simulink model "power_aircraft_distribution_mexido_2016_V4"  (R2016a)
settings: Solver=ode23t  StartTime=72.95  StopTime=73.6  MaxStep=0.01  RelTol=0.5e-4  AbsTol=0.5e-4
PreLoadFcn:
  | % -- Recommended Settings --
  | %
  | %  Simulink:
  | %      Solver: Ode23t
  | %      Relative tolerance = 1e-3
  | %       Max step size = 0.2
  | %
  | %  Powergui:
  |          Ts = 1e-07; % (discrete electrical model)
  | %
  | %  Control systems:
  |          Ts_control = 10*Ts; % (discrete control system)
  | %
  | % ----------------------------------
undefined symbols (not defined in the file or in its folder): C, D1, Delta, L, sigbuilder_block, tb1, tb2, tb3
libraries: powerlib x79, dsparch4 x12, simulink x6, sps_avr x1, powerlib_meascontrol x1
(part 1 of 2)
settings Model: Creator=Joao  LastModifiedBy=Joao
settings DataIOCC: InitialState=xFinal  LimitDataPoints=on  SaveCompleteFinalSimState=on
settings DebuggingCC: AllowSymbolicDim=off
settings ConfigComp: CovModelRefEnable=Off  CovSFcnEnable=off

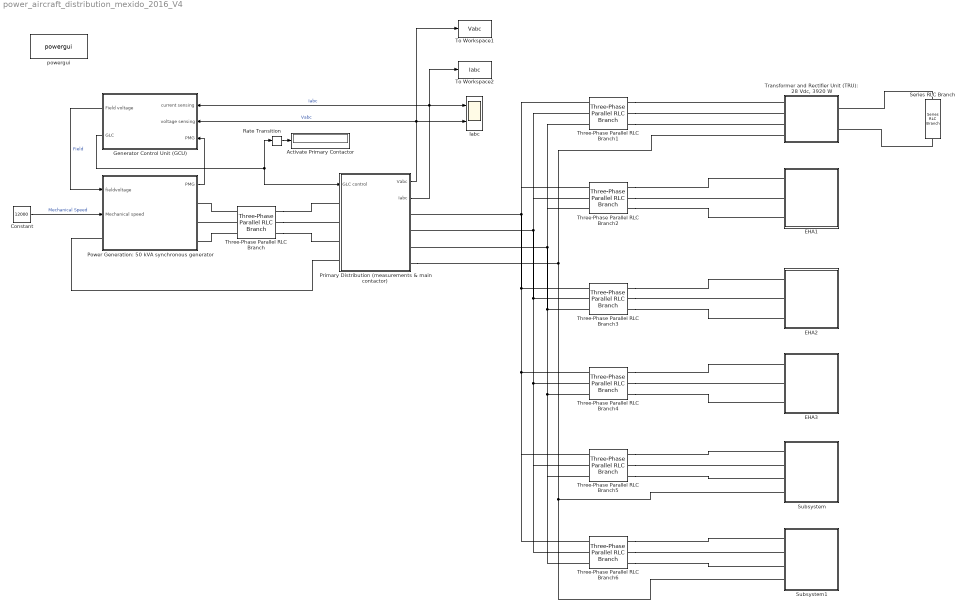
== system power_aircraft_distribution_mexido_2016_V4 ==
  Activate Primary Contactor : Display
      settings: SampleTime=1e-2
  Constant : Constant  Value=12000
  EHA1 : Subsystem
  EHA2 : Subsystem
  EHA3 : Subsystem
  Generator Control Unit (GCU) : Subsystem
      mask Display: image(imread('power_aircraft_distribution_GCU.jpg','jpg'))
  Iabc : Scope  NumInputPorts=2
  Power Generation: 50 kVA synchronous generator : Subsystem
      mask Display: image(imread('power_aircraft_distribution_APU_Generator.jpg','jpg'))
  Primary Distribution (measurements & main contactor) : Subsystem
  Rate Transition : RateTransition  OutPortSampleTimeOpt=Inherit  OutPortSampleTime=Ts
  Series RLC Branch : powerlib/Elements/Series RLC Branch  LConnTagsString=__new0  RConnTagsString=__new0  BranchType=R  Resistance=0.2  Inductance=1e-3  SetiL0=off  InitialCurrent=0  Capacitance=1e-6  Setx0=off  InitialVoltage=0  Measurements=None
  Subsystem : Subsystem
  Subsystem1 : Subsystem
  Three-Phase Parallel RLC Branch : powerlib/Elements/Three-Phase Parallel RLC Branch  LConnTagsString=A|B|C  RConnTagsString=A|B|C  BranchType=RL  Resistance=0.00047*10  Inductance=5e-6  Capacitance=0  Measurements=None
  Three-Phase Parallel RLC Branch1 : powerlib/Elements/Three-Phase Parallel RLC Branch  LConnTagsString=A|B|C  RConnTagsString=A|B|C  BranchType=RL  Resistance=0.00228*3  Inductance=5e-7  Capacitance=0  Measurements=None
  Three-Phase Parallel RLC Branch2 : powerlib/Elements/Three-Phase Parallel RLC Branch  LConnTagsString=A|B|C  RConnTagsString=A|B|C  BranchType=RL  Resistance=0.00227*15  Inductance=3e-6  Capacitance=0  Measurements=None
  Three-Phase Parallel RLC Branch3 : powerlib/Elements/Three-Phase Parallel RLC Branch  LConnTagsString=A|B|C  RConnTagsString=A|B|C  BranchType=RL  Resistance=0.00227*17.5  Inductance=3e-6  Capacitance=0  Measurements=None
  Three-Phase Parallel RLC Branch4 : powerlib/Elements/Three-Phase Parallel RLC Branch  LConnTagsString=A|B|C  RConnTagsString=A|B|C  BranchType=RL  Resistance=0.00227*20  Inductance=3e-6  Capacitance=0  Measurements=None
  Three-Phase Parallel RLC Branch5 : powerlib/Elements/Three-Phase Parallel RLC Branch  LConnTagsString=A|B|C  RConnTagsString=A|B|C  BranchType=RL  Resistance=0.00228*20  Inductance=10e-6  Capacitance=0  Measurements=None
  Three-Phase Parallel RLC Branch6 : powerlib/Elements/Three-Phase Parallel RLC Branch  LConnTagsString=A|B|C  RConnTagsString=A|B|C  BranchType=RL  Resistance=0.00228*8  Inductance=5e-6  Capacitance=0  Measurements=None
  To Workspace1 : ToWorkspace  VariableName=Vabc  SaveFormat=Structure With Time  SampleTime=-1
  To Workspace2 : ToWorkspace  VariableName=Iabc  SaveFormat=Structure With Time  SampleTime=-1
  "Transformer and Rectifier Unit (TRU): 28 Vdc, 3920 W" : Subsystem
      mask Display: image(imread('power_aircraft_distribution_TRU.jpg','jpg'))
  powergui : powerlib/powergui  Priority=1  SimulationMode=Discrete  SolverType=Tustin/Backward Euler (TBE)  SampleTime=Ts  frequency=60  SPID=off  DisableSnubberDevices=off  DisableRonSwitches=off  DisableVfSwitches=off  SwTol=0  DisplayEquations=off  Interpol=off  ExternalGateDelay=off  methode=off  Ts=100  FunctionMessages=on  echomessages=off  HookPort=off  EnableUseOfTLC=off  x0status=blocks  frequencyindice=0  Pbase=100e6  ErrMax=1e-4  Iterations=50  UnitsV=kV  UnitsW=MW  buscounter=0  RestoreLinks=warning  ResistiveCurrentMeasurement=off  Frange=[0:2:500]  Ylog=off  Xlog=on  ShowGrid=off  save=off  variable=ZData  structure=0  ZoomFFT=off  StartTime=0.0  cycles=1  DisplayStyle=1  fundamental=60  FreqAxis=off  MaxFrequency=1000  frequencyindicesteady=1  RmsSteady=1  display=off
  wires:
  Power Generation: 50 kVA synchronous generator/1(PMG) -> Generator Control Unit (GCU)/3(PMG)
  Generator Control Unit (GCU)/1(Field voltage) -> Power Generation: 50 kVA synchronous generator/1(fieldvoltage)  "Field"
  Primary Distribution (measurements & main contactor)/1(Vabc) -> Generator Control Unit (GCU)/2(voltage sensing), To Workspace1/1, Iabc/2  "Vabc"
  Primary Distribution (measurements & main contactor)/2(Iabc) -> To Workspace2/1, Generator Control Unit (GCU)/1(current sensing), Iabc/1  "Iabc"
  Generator Control Unit (GCU)/2(GLC) -> Primary Distribution (measurements & main contactor)/1(GLC control), Rate Transition/1
  Constant/1 -> Power Generation: 50 kVA synchronous generator/2(Mechanical speed)  "Mechanical Speed"
  Rate Transition/1 -> Activate Primary Contactor/1
  connections:
  Three-Phase Parallel RLC Branch6/LConn1 -- Three-Phase Parallel RLC Branch5/LConn1 -- Three-Phase Parallel RLC Branch4/LConn1 -- Three-Phase Parallel RLC Branch3/LConn1 -- Primary Distribution (measurements & main contactor)/RConn1 -- Three-Phase Parallel RLC Branch2/LConn1 -- Three-Phase Parallel RLC Branch1/LConn1
  Primary Distribution (measurements & main contactor)/RConn4 -- "Transformer and Rectifier Unit (TRU): 28 Vdc, 3920 W"/LConn4 -- Subsystem1/LConn4 -- Subsystem/LConn4
  Three-Phase Parallel RLC Branch6/LConn3 -- Three-Phase Parallel RLC Branch5/LConn3 -- Three-Phase Parallel RLC Branch4/LConn3 -- Three-Phase Parallel RLC Branch3/LConn3 -- Primary Distribution (measurements & main contactor)/RConn3 -- Three-Phase Parallel RLC Branch2/LConn3 -- Three-Phase Parallel RLC Branch1/LConn3
  Three-Phase Parallel RLC Branch6/LConn2 -- Three-Phase Parallel RLC Branch5/LConn2 -- Three-Phase Parallel RLC Branch4/LConn2 -- Three-Phase Parallel RLC Branch3/LConn2 -- Primary Distribution (measurements & main contactor)/RConn2 -- Three-Phase Parallel RLC Branch2/LConn2 -- Three-Phase Parallel RLC Branch1/LConn2
  Three-Phase Parallel RLC Branch/RConn2 -- Primary Distribution (measurements & main contactor)/LConn2
  Three-Phase Parallel RLC Branch/LConn2 -- Power Generation: 50 kVA synchronous generator/RConn2
  Three-Phase Parallel RLC Branch/LConn1 -- Power Generation: 50 kVA synchronous generator/RConn1
  Three-Phase Parallel RLC Branch/LConn3 -- Power Generation: 50 kVA synchronous generator/RConn3
  Three-Phase Parallel RLC Branch/RConn1 -- Primary Distribution (measurements & main contactor)/LConn1
  Three-Phase Parallel RLC Branch/RConn3 -- Primary Distribution (measurements & main contactor)/LConn3
  Power Generation: 50 kVA synchronous generator/LConn1 -- Primary Distribution (measurements & main contactor)/LConn4
  Series RLC Branch/RConn1 -- "Transformer and Rectifier Unit (TRU): 28 Vdc, 3920 W"/RConn2
  Series RLC Branch/LConn1 -- "Transformer and Rectifier Unit (TRU): 28 Vdc, 3920 W"/RConn1
  Three-Phase Parallel RLC Branch1/RConn1 -- "Transformer and Rectifier Unit (TRU): 28 Vdc, 3920 W"/LConn1
  Three-Phase Parallel RLC Branch1/RConn2 -- "Transformer and Rectifier Unit (TRU): 28 Vdc, 3920 W"/LConn2
  Three-Phase Parallel RLC Branch1/RConn3 -- "Transformer and Rectifier Unit (TRU): 28 Vdc, 3920 W"/LConn3
  Three-Phase Parallel RLC Branch5/RConn1 -- Subsystem/LConn1
  Three-Phase Parallel RLC Branch5/RConn2 -- Subsystem/LConn2
  Three-Phase Parallel RLC Branch5/RConn3 -- Subsystem/LConn3
  Three-Phase Parallel RLC Branch6/RConn1 -- Subsystem1/LConn1
  Three-Phase Parallel RLC Branch6/RConn2 -- Subsystem1/LConn2
  Three-Phase Parallel RLC Branch6/RConn3 -- Subsystem1/LConn3
  Three-Phase Parallel RLC Branch2/RConn1 -- EHA1/LConn1
  Three-Phase Parallel RLC Branch2/RConn2 -- EHA1/LConn2
  Three-Phase Parallel RLC Branch2/RConn3 -- EHA1/LConn3
  Three-Phase Parallel RLC Branch3/RConn1 -- EHA2/LConn1
  Three-Phase Parallel RLC Branch3/RConn2 -- EHA2/LConn2
  Three-Phase Parallel RLC Branch3/RConn3 -- EHA2/LConn3
  Three-Phase Parallel RLC Branch4/RConn1 -- EHA3/LConn1
  Three-Phase Parallel RLC Branch4/RConn2 -- EHA3/LConn2
  Three-Phase Parallel RLC Branch4/RConn3 -- EHA3/LConn3

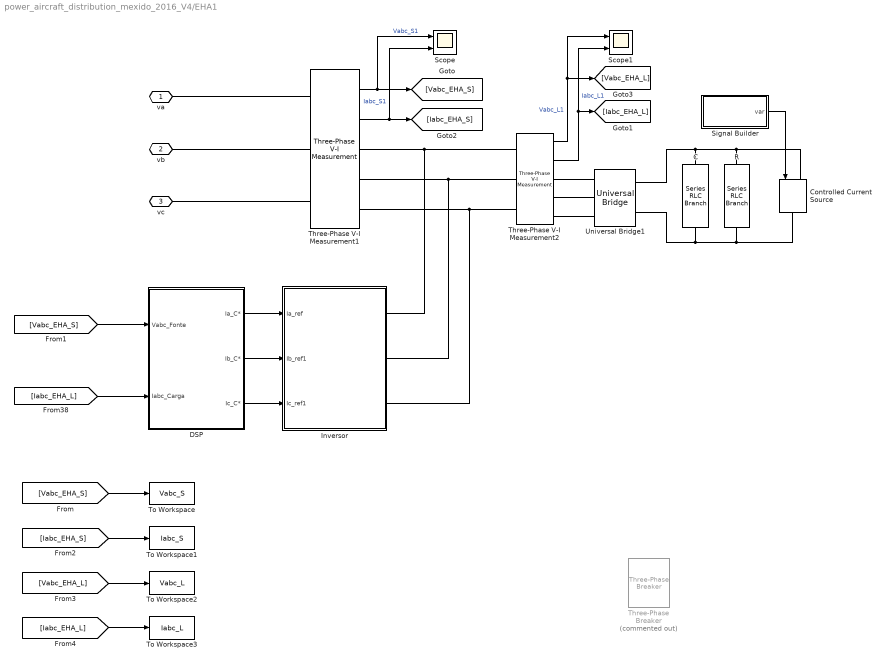
== system power_aircraft_distribution_mexido_2016_V4/EHA1 ==
  C : powerlib/Elements/Series RLC Branch  LConnTagsString=__new0  RConnTagsString=__new0  BranchType=C  Resistance=1  Inductance=1e-3  SetiL0=off  InitialCurrent=0  Capacitance=1e-7  Setx0=off  InitialVoltage=0  Measurements=None
  Controlled Current Source : powerlib/Electrical Sources/Controlled Current Source  Initialize=on  Source_Type=AC  Amplitude=0  Phase=0  Frequency=0  Measurements=None
  DSP : Subsystem
  Inversor : Subsystem
  R : powerlib/Elements/Series RLC Branch  LConnTagsString=__new0  RConnTagsString=__new0  BranchType=R  Resistance=400  Inductance=1e-3  SetiL0=off  InitialCurrent=0  Capacitance=1e-10  Setx0=off  InitialVoltage=0  Measurements=None
  Scope : Scope  NumInputPorts=2
  Scope1 : Scope  NumInputPorts=2
  Signal Builder : Subsystem  Tag=STV Subsys  LoadFcn=sigbuilder_block('load',[437.6 199.2 550.4 400 ]);  StartFcn=sigbuilder_block('start');  StopFcn=sigbuilder_block('stop');  ClipboardFcn=sigbuilder_block('clipboard');  mask(Sigbuilder block){}
      mask help: Simulink:masks:SigbuilderBlock_MD
      mask init:
      | if ~strcmp(get_param(bdroot(gcbh),'SimulationStatus'),'stopped') tuvar = sigbuilder_block('maskInit'); end
      settings: CopyFcn=sigbuilder_block('copy');  DeleteFcn=sigbuilder_block('delete');  ModelCloseFcn=sigbuilder_block('modelClose');  PreSaveFcn=sigbuilder_block('preSave');  PauseFcn=sigbuilder_block('pause');  ContinueFcn=sigbuilder_block('continue');  NameChangeFcn=sigbuilder_block('namechange');  OpenFcn=sigbuilder_block('open',[437.6 199.2 550.4 400 ]);  CloseFcn=sigbuilder_block('close');
      mask Display: plot(0, 0, 100, 100,[2, 2, 32, 32, 2], [68, 8, 8, 68, 68],[32, 2], [38, 38], [32, 19, 2],[53, 60, 44], [32, 17, 17, 2],[16, 16, 31, 31]);txt = getActiveGroup(gcbh);text(2, 100, txt,'verticalAlignment', 'top');
  Three-Phase V-I Measurement1 : powerlib/Measurements/Three-Phase V-I Measurement  VoltageMeasurement=phase-to-ground  SetLabelV=off  LabelV=Vabc_EHA1_S  Vpu=off  VpuLL=off  CurrentMeasurement=yes  SetLabelI=off  LabelI=Iabc_EHA1_S  Ipu=off  Pbase=100e6  Vbase=500e3  OutputType=Complex  PhasorSimulation=off  PSBequivalent=0
  Three-Phase V-I Measurement2 : powerlib/Measurements/Three-Phase V-I Measurement  VoltageMeasurement=phase-to-ground  SetLabelV=off  LabelV=Vabc_EHA1_S  Vpu=off  VpuLL=off  CurrentMeasurement=yes  SetLabelI=off  LabelI=Iabc_EHA1_S  Ipu=off  Pbase=100e6  Vbase=500e3  OutputType=Complex  PhasorSimulation=off  PSBequivalent=0
  Three-Phase Breaker : powerlib/Elements/Three-Phase Breaker  Commented=on  InitialState=open  SwitchA=on  SwitchB=on  SwitchC=on  SwitchTimes=tb1  External=off  BreakerResistance=1e-3  SnubberResistance=1e6  SnubberCapacitance=inf  Measurements=None
  To Workspace : ToWorkspace  VariableName=Vabc_S  SaveFormat=Structure With Time  SampleTime=-1
  To Workspace1 : ToWorkspace  VariableName=Iabc_S  SaveFormat=Structure With Time  SampleTime=-1
  To Workspace2 : ToWorkspace  VariableName=Vabc_L  SaveFormat=Structure With Time  SampleTime=-1
  To Workspace3 : ToWorkspace  VariableName=Iabc_L  SaveFormat=Structure With Time  SampleTime=-1
  Universal Bridge1 : powerlib/Power Electronics/Universal Bridge  Arms=3  SnubberResistance=1e5  SnubberCapacitance=inf  Device=Diodes  Ron=1e-9  Lon=0  ForwardVoltages="[  0  0  ]"  ForwardVoltage=0  GTOparameters=[ 10e-6 , 20e-6 ]  IGBTparameters=[ 1e-6 , 2e-6 ]  Measurements=None  Measurements_2=None  converterType=Rectifier
  va : PMIOPort  Port=1  Side=Left
  vb : PMIOPort  Port=2  Side=Left
  vc : PMIOPort  Port=3  Side=Left
  wires:
  Signal Builder/1(var) -> Controlled Current Source/1
  Three-Phase V-I Measurement1/1 -> [Vabc_EHA_S], Scope/1  "Vabc_S1"
  Three-Phase V-I Measurement1/2 -> [Iabc_EHA_S], Scope/2  "Iabc_S1"
  Three-Phase V-I Measurement2/1 -> [Vabc_EHA_L], Scope1/1  "Vabc_L1"
  Three-Phase V-I Measurement2/2 -> [Iabc_EHA_L], Scope1/2  "Iabc_L1"
  [Vabc_EHA_S] -> DSP/1(Vabc_Fonte)
  [Iabc_EHA_L] -> DSP/2(Iabc_Carga)
  DSP/1(Ia_C*) -> Inversor/1(Ia_ref)
  DSP/2(Ib_C*) -> Inversor/2(Ib_ref1)
  DSP/3(Ic_C*) -> Inversor/3(Ic_ref1)
  [Vabc_EHA_S] -> To Workspace/1
  [Iabc_EHA_S] -> To Workspace1/1
  [Vabc_EHA_L] -> To Workspace2/1
  [Iabc_EHA_L] -> To Workspace3/1
  connections:
  R/LConn1 -- Controlled Current Source/LConn1 -- Universal Bridge1/RConn1 -- C/LConn1
  Controlled Current Source/RConn1 -- R/RConn1 -- Universal Bridge1/RConn2 -- C/RConn1
  Three-Phase V-I Measurement2/RConn2 -- Universal Bridge1/LConn2
  Three-Phase V-I Measurement2/RConn1 -- Universal Bridge1/LConn1
  Three-Phase V-I Measurement2/RConn3 -- Universal Bridge1/LConn3
  Three-Phase V-I Measurement1/RConn3 -- Three-Phase V-I Measurement2/LConn3 -- Inversor/RConn3
  Three-Phase V-I Measurement2/LConn1 -- Three-Phase V-I Measurement1/RConn1 -- Inversor/RConn1
  Three-Phase V-I Measurement2/LConn2 -- Three-Phase V-I Measurement1/RConn2 -- Inversor/RConn2
  vb/RConn1 -- Three-Phase V-I Measurement1/LConn2
  vc/RConn1 -- Three-Phase V-I Measurement1/LConn3
  va/RConn1 -- Three-Phase V-I Measurement1/LConn1

== system power_aircraft_distribution_mexido_2016_V4/EHA2 ==
  C : powerlib/Elements/Series RLC Branch  LConnTagsString=__new0  RConnTagsString=__new0  BranchType=C  Resistance=1  Inductance=1e-3  SetiL0=off  InitialCurrent=0  Capacitance=1e-7  Setx0=off  InitialVoltage=0  Measurements=None
  Controlled Current Source : powerlib/Electrical Sources/Controlled Current Source  Initialize=on  Source_Type=AC  Amplitude=0  Phase=0  Frequency=0  Measurements=None
  DSP : Subsystem
  Inversor : Subsystem
  R : powerlib/Elements/Series RLC Branch  LConnTagsString=__new0  RConnTagsString=__new0  BranchType=R  Resistance=400  Inductance=1e-3  SetiL0=off  InitialCurrent=0  Capacitance=1e-10  Setx0=off  InitialVoltage=0  Measurements=None
  Scope : Scope  NumInputPorts=2
  Scope1 : Scope  NumInputPorts=2
  Signal Builder : Subsystem  Tag=STV Subsys  LoadFcn=sigbuilder_block('load');  StartFcn=sigbuilder_block('start');  StopFcn=sigbuilder_block('stop');  ClipboardFcn=sigbuilder_block('clipboard');  mask(Sigbuilder block){}
      mask help: Simulink:masks:SigbuilderBlock_MD
      mask init:
      | if ~strcmp(get_param(bdroot(gcbh),'SimulationStatus'),'stopped') tuvar = sigbuilder_block('maskInit'); end
      settings: CopyFcn=sigbuilder_block('copy');  DeleteFcn=sigbuilder_block('delete');  ModelCloseFcn=sigbuilder_block('modelClose');  PreSaveFcn=sigbuilder_block('preSave');  PauseFcn=sigbuilder_block('pause');  ContinueFcn=sigbuilder_block('continue');  NameChangeFcn=sigbuilder_block('namechange');  OpenFcn=sigbuilder_block('open',[437.6 199.2 550.4 400 ]);  CloseFcn=sigbuilder_block('close');
      mask Display: plot(0, 0, 100, 100,[2, 2, 32, 32, 2], [68, 8, 8, 68, 68],[32, 2], [38, 38], [32, 19, 2],[53, 60, 44], [32, 17, 17, 2],[16, 16, 31, 31]);txt = getActiveGroup(gcbh);text(2, 100, txt,'verticalAlignment', 'top');
  Three-Phase V-I Measurement1 : powerlib/Measurements/Three-Phase V-I Measurement  VoltageMeasurement=phase-to-ground  SetLabelV=off  LabelV=Vabc_EHA1_S  Vpu=off  VpuLL=off  CurrentMeasurement=yes  SetLabelI=off  LabelI=Iabc_EHA1_S  Ipu=off  Pbase=100e6  Vbase=500e3  OutputType=Complex  PhasorSimulation=off  PSBequivalent=0
  Three-Phase V-I Measurement2 : powerlib/Measurements/Three-Phase V-I Measurement  VoltageMeasurement=phase-to-ground  SetLabelV=off  LabelV=Vabc_EHA1_S  Vpu=off  VpuLL=off  CurrentMeasurement=yes  SetLabelI=off  LabelI=Iabc_EHA1_S  Ipu=off  Pbase=100e6  Vbase=500e3  OutputType=Complex  PhasorSimulation=off  PSBequivalent=0
  Three-Phase Breaker : powerlib/Elements/Three-Phase Breaker  Commented=on  InitialState=open  SwitchA=on  SwitchB=on  SwitchC=on  SwitchTimes=tb2  External=off  BreakerResistance=1e-3  SnubberResistance=1e6  SnubberCapacitance=inf  Measurements=None
  Universal Bridge1 : powerlib/Power Electronics/Universal Bridge  Arms=3  SnubberResistance=1e5  SnubberCapacitance=inf  Device=Diodes  Ron=1e-9  Lon=0  ForwardVoltages="[  0  0  ]"  ForwardVoltage=0  GTOparameters=[ 10e-6 , 20e-6 ]  IGBTparameters=[ 1e-6 , 2e-6 ]  Measurements=None  Measurements_2=None  converterType=Rectifier
  va : PMIOPort  Port=1  Side=Left
  vb : PMIOPort  Port=2  Side=Left
  vc : PMIOPort  Port=3  Side=Left
  wires:
  Signal Builder/1(var) -> Controlled Current Source/1
  Three-Phase V-I Measurement1/1 -> [Vabc_EHA_S], Scope/1  "Vabc_S2"
  Three-Phase V-I Measurement1/2 -> Scope/2  "Iabc_S2"
  Three-Phase V-I Measurement2/1 -> Scope1/1  "Vabc_L2"
  Three-Phase V-I Measurement2/2 -> [Iabc_EHA_L], Scope1/2  "Iabc_L2"
  [Vabc_EHA_S] -> DSP/1(Vabc_Fonte)
  [Iabc_EHA_L] -> DSP/2(Iabc_Carga)
  DSP/1(Ia_C*) -> Inversor/1(Ia_ref)
  DSP/2(Ib_C*) -> Inversor/2(Ib_ref1)
  DSP/3(Ic_C*) -> Inversor/3(Ic_ref1)
  connections:
  R/LConn1 -- Controlled Current Source/LConn1 -- Universal Bridge1/RConn1 -- C/LConn1
  Controlled Current Source/RConn1 -- R/RConn1 -- Universal Bridge1/RConn2 -- C/RConn1
  Three-Phase V-I Measurement2/RConn2 -- Universal Bridge1/LConn2
  Three-Phase V-I Measurement2/RConn1 -- Universal Bridge1/LConn1
  Three-Phase V-I Measurement2/RConn3 -- Universal Bridge1/LConn3
  Three-Phase V-I Measurement1/RConn3 -- Three-Phase V-I Measurement2/LConn3 -- Inversor/RConn3
  Three-Phase V-I Measurement2/LConn1 -- Three-Phase V-I Measurement1/RConn1 -- Inversor/RConn1
  Three-Phase V-I Measurement2/LConn2 -- Three-Phase V-I Measurement1/RConn2 -- Inversor/RConn2
  Three-Phase V-I Measurement1/LConn2 -- vb/RConn1
  vc/RConn1 -- Three-Phase V-I Measurement1/LConn3
  va/RConn1 -- Three-Phase V-I Measurement1/LConn1

== system power_aircraft_distribution_mexido_2016_V4/EHA3 ==
  C : powerlib/Elements/Series RLC Branch  LConnTagsString=__new0  RConnTagsString=__new0  BranchType=C  Resistance=1  Inductance=1e-3  SetiL0=off  InitialCurrent=0  Capacitance=1e-7  Setx0=off  InitialVoltage=0  Measurements=None
  Controlled Current Source : powerlib/Electrical Sources/Controlled Current Source  Initialize=on  Source_Type=AC  Amplitude=0  Phase=0  Frequency=0  Measurements=None
  DSP : Subsystem
  Inversor : Subsystem
  R : powerlib/Elements/Series RLC Branch  LConnTagsString=__new0  RConnTagsString=__new0  BranchType=R  Resistance=400  Inductance=1e-3  SetiL0=off  InitialCurrent=0  Capacitance=1e-10  Setx0=off  InitialVoltage=0  Measurements=None
  Scope : Scope  NumInputPorts=2
  Scope1 : Scope  NumInputPorts=2
  Signal Builder : Subsystem  Tag=STV Subsys  LoadFcn=sigbuilder_block('load');  StartFcn=sigbuilder_block('start');  StopFcn=sigbuilder_block('stop');  ClipboardFcn=sigbuilder_block('clipboard');  mask(Sigbuilder block){}
      mask help: Simulink:masks:SigbuilderBlock_MD
      mask init:
      | if ~strcmp(get_param(bdroot(gcbh),'SimulationStatus'),'stopped') tuvar = sigbuilder_block('maskInit'); end
      settings: CopyFcn=sigbuilder_block('copy');  DeleteFcn=sigbuilder_block('delete');  ModelCloseFcn=sigbuilder_block('modelClose');  PreSaveFcn=sigbuilder_block('preSave');  PauseFcn=sigbuilder_block('pause');  ContinueFcn=sigbuilder_block('continue');  NameChangeFcn=sigbuilder_block('namechange');  OpenFcn=sigbuilder_block('open',[437.6 199.2 550.4 400 ]);  CloseFcn=sigbuilder_block('close');
      mask Display: plot(0, 0, 100, 100,[2, 2, 32, 32, 2], [68, 8, 8, 68, 68],[32, 2], [38, 38], [32, 19, 2],[53, 60, 44], [32, 17, 17, 2],[16, 16, 31, 31]);txt = getActiveGroup(gcbh);text(2, 100, txt,'verticalAlignment', 'top');
  Three-Phase V-I Measurement1 : powerlib/Measurements/Three-Phase V-I Measurement  VoltageMeasurement=phase-to-ground  SetLabelV=off  LabelV=Vabc_EHA1_S  Vpu=off  VpuLL=off  CurrentMeasurement=yes  SetLabelI=off  LabelI=Iabc_EHA1_S  Ipu=off  Pbase=100e6  Vbase=500e3  OutputType=Complex  PhasorSimulation=off  PSBequivalent=0
  Three-Phase V-I Measurement2 : powerlib/Measurements/Three-Phase V-I Measurement  VoltageMeasurement=phase-to-ground  SetLabelV=off  LabelV=Vabc_EHA1_S  Vpu=off  VpuLL=off  CurrentMeasurement=yes  SetLabelI=off  LabelI=Iabc_EHA1_S  Ipu=off  Pbase=100e6  Vbase=500e3  OutputType=Complex  PhasorSimulation=off  PSBequivalent=0
  Three-Phase Breaker : powerlib/Elements/Three-Phase Breaker  Commented=on  InitialState=open  SwitchA=on  SwitchB=on  SwitchC=on  SwitchTimes=tb3  External=off  BreakerResistance=1e-3  SnubberResistance=1e6  SnubberCapacitance=inf  Measurements=None
  Universal Bridge1 : powerlib/Power Electronics/Universal Bridge  Arms=3  SnubberResistance=1e5  SnubberCapacitance=inf  Device=Diodes  Ron=1e-9  Lon=0  ForwardVoltages="[  0  0  ]"  ForwardVoltage=0  GTOparameters=[ 10e-6 , 20e-6 ]  IGBTparameters=[ 1e-6 , 2e-6 ]  Measurements=None  Measurements_2=None  converterType=Rectifier
  va : PMIOPort  Port=1  Side=Left
  vb : PMIOPort  Port=2  Side=Left
  vc : PMIOPort  Port=3  Side=Left
  wires:
  Signal Builder/1(var) -> Controlled Current Source/1
  Three-Phase V-I Measurement1/1 -> [Vabc_EHA_S], Scope/1  "Vabc_S3"
  Three-Phase V-I Measurement1/2 -> Scope/2  "Iabc_S3"
  Three-Phase V-I Measurement2/1 -> Scope1/1  "Vabc_L3"
  Three-Phase V-I Measurement2/2 -> [Iabc_EHA_L], Scope1/2  "Iabc_L3"
  [Vabc_EHA_S] -> DSP/1(Vabc_Fonte)
  [Iabc_EHA_L] -> DSP/2(Iabc_Carga)
  DSP/1(Ia_C*) -> Inversor/1(Ia_ref)
  DSP/2(Ib_C*) -> Inversor/2(Ib_ref1)
  DSP/3(Ic_C*) -> Inversor/3(Ic_ref1)
  connections:
  R/LConn1 -- Controlled Current Source/LConn1 -- Universal Bridge1/RConn1 -- C/LConn1
  Controlled Current Source/RConn1 -- R/RConn1 -- Universal Bridge1/RConn2 -- C/RConn1
  Three-Phase V-I Measurement2/RConn2 -- Universal Bridge1/LConn2
  Three-Phase V-I Measurement2/RConn1 -- Universal Bridge1/LConn1
  Three-Phase V-I Measurement2/RConn3 -- Universal Bridge1/LConn3
  Three-Phase V-I Measurement1/RConn3 -- Three-Phase V-I Measurement2/LConn3 -- Inversor/RConn3
  Three-Phase V-I Measurement2/LConn1 -- Three-Phase V-I Measurement1/RConn1 -- Inversor/RConn1
  Three-Phase V-I Measurement2/LConn2 -- Three-Phase V-I Measurement1/RConn2 -- Inversor/RConn2
  vc/RConn1 -- Three-Phase V-I Measurement1/LConn3
  va/RConn1 -- Three-Phase V-I Measurement1/LConn1
  vb/RConn1 -- Three-Phase V-I Measurement1/LConn2

== system power_aircraft_distribution_mexido_2016_V4/Generator Control Unit (GCU) ==
  current sensing : Inport
  voltage sensing : Inport  Port=2
  PMG : Inport  Port=3
  Demux : Demux  Outputs=3
  Excitation System : sps_avr/Excitation System  tr=20e-3  reg=[ 300, 0.001 ]  exc=[ 1, 0 ]  tgr=[ 0, 0 ]  damp=[ 0.001, 0.1 ]  sat=[ 0, 0 ]  lim=[ -2, 2, 0 ]  v0=[1 0]
  Gain : Gain  Gain=2
  Integrator : Integrator
  PU_SI : Gain  Gain=200
  Rad_Rpm : Gain  Gain=30/pi
  Relay : Relay  OnSwitchValue=9000  OffSwitchValue=8900
  SI_PU : Gain  Gain=1/(115*sqrt(2))
  Terminator1 : Terminator
  Terminator2 : Terminator
  Vref : Constant
  abc to dq0 : powerlib_meascontrol/Transformations/abc to dq0  Alignment=90 degrees behind phase A axis
  threshold3 : Constant  Value=0
  Field voltage : Outport
  GLC : Outport  Port=2
  wires:
  Relay/1 -> GLC/1
  Demux/3 -> Terminator2/1
  current sensing/1 -> Terminator1/1
  threshold3/1 -> Excitation System/4
  Vref/1 -> Excitation System/1
  Rad_Rpm/1 -> Relay/1
  PU_SI/1 -> Field voltage/1
  Excitation System/1 -> PU_SI/1
  SI_PU/1 -> abc to dq0/1
  Demux/2 -> Excitation System/3
  Demux/1 -> Excitation System/2
  abc to dq0/1 -> Demux/1
  Integrator/1 -> Gain/1
  voltage sensing/1 -> SI_PU/1
  PMG/1 -> Rad_Rpm/1, Integrator/1
  Gain/1 -> abc to dq0/2

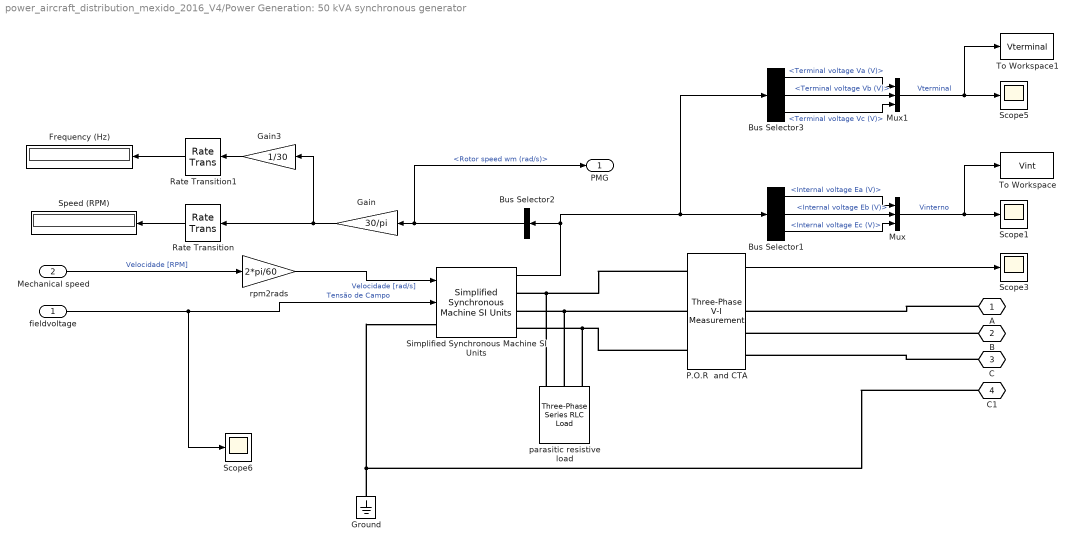
== system power_aircraft_distribution_mexido_2016_V4/Power Generation: 50 kVA synchronous generator ==
  fieldvoltage : Inport
  Mechanical speed : Inport  Port=2
  Bus Selector1 : BusSelector  OutputSignals=Internal voltage Ea (V),Internal voltage Eb (V),Internal voltage Ec (V)
  Bus Selector2 : BusSelector  OutputSignals=Rotor speed wm (rad/s)
  Bus Selector3 : BusSelector  OutputSignals=Terminal voltage Va (V),Terminal voltage Vb (V),Terminal voltage Vc (V)
  Frequency (Hz) : Display
      settings: SampleTime=1e-2
  Gain : Gain  Gain=30/pi
  Gain3 : Gain  Gain=1/30
  Ground : powerlib/Elements/Ground  LConnTagsString=a
  Mux : Mux  Inputs=3
  Mux1 : Mux  Inputs=3
  P.O.R  and CTA : powerlib/Measurements/Three-Phase V-I Measurement  VoltageMeasurement=phase-to-ground  SetLabelV=off  LabelV=Vabc  Vpu=off  VpuLL=off  CurrentMeasurement=yes  SetLabelI=off  LabelI=Iabc  Ipu=off  Pbase=100e6  Vbase=500e3  OutputType=Complex  PhasorSimulation=off  PSBequivalent=0
  Rate Transition : RateTransition  OutPortSampleTimeOpt=Inherit  OutPortSampleTime=Ts
  Rate Transition1 : RateTransition  OutPortSampleTimeOpt=Inherit  OutPortSampleTime=Ts
  Scope{1,3,5..6} (4 alike) : Scope
  Simplified Synchronous Machine SI Units : powerlib/Machines/Simplified Synchronous Machine SI Units  ConnectionType=4-wire Y  MechanicalLoad=Speed w  MeasurementBus=off  NominalParameters=[50e3 200 400]  Mechanical=[0.02 0 2]  InternalRL="[0.0204  0.08104e-3]"  InitialConditions=[-99,0 0,0,0 0,0,0]  Units=1  LoadFlowParameters=[1,0,0,0,0]  TsPowergui=0  TsBlock=Ts  BusType=PV  Pref=0  Qref=0  Qmin=-inf  Qmax=+inf  PLF=0  QLF=0
  Speed (RPM) : Display
      settings: SampleTime=1e-2
  To Workspace : ToWorkspace  VariableName=Vint  SaveFormat=Structure With Time  SampleTime=-1
  To Workspace1 : ToWorkspace  VariableName=Vterminal  SaveFormat=Structure With Time  SampleTime=-1
  parasitic resistive load : powerlib/Elements/Three-Phase Series RLC Load  LConnTagsString=A|B|C  Configuration=Y (grounded)  NominalVoltage=200  Vabc=[1e3 1e3 1e3]  Vabcp=[1e3 1e3 1e3]  NominalFrequency=400  UnbalancedPower=off  ActivePower=5000  InductivePower=0  CapacitivePower=0  Pabc=[10e3 9e3 11e3]  QLabc=[100 90 110]  QCabc=[100 90 110]  Pabcp=[10e3 9e3 11e3]  QLabcp=[100 90 110]  QCabcp=[100 90 110]  Measurements=None  LoadType=constant Z
  rpm2rads : Gain  Gain=2*pi/60
  A : PMIOPort  Tag=PMCPort  Port=1  Side=Right
  B : PMIOPort  Tag=PMCPort  Port=2  Side=Right
  C : PMIOPort  Tag=PMCPort  Port=3  Side=Right
  C1 : PMIOPort  Tag=PMCPort  Port=4  Side=Left
  PMG : Outport
  wires:
  Simplified Synchronous Machine SI Units/1 -> Bus Selector3/1, Bus Selector1/1, Bus Selector2/1
  fieldvoltage/1 -> Scope6/1, Simplified Synchronous Machine SI Units/2  "Tensão de Campo"
  Bus Selector2/1 -> PMG/1, Gain/1  "<Rotor speed wm (rad/s)>"
  Gain/1 -> Gain3/1, Rate Transition/1
  Gain3/1 -> Rate Transition1/1
  Mechanical speed/1 -> rpm2rads/1  "Velocidade [RPM]"
  rpm2rads/1 -> Simplified Synchronous Machine SI Units/1  "Velocidade [rad/s]"
  Rate Transition/1 -> Speed (RPM)/1
  Rate Transition1/1 -> Frequency (Hz)/1
  Bus Selector1/2 -> Mux/2  "<Internal voltage Eb (V)>"
  Bus Selector1/3 -> Mux/3  "<Internal voltage Ec (V)>"
  Bus Selector1/1 -> Mux/1  "<Internal voltage Ea (V)>"
  Mux/1 -> Scope1/1, To Workspace/1  "Vinterno"
  P.O.R  and CTA/1 -> Scope3/1
  Bus Selector3/2 -> Mux1/2  "<Terminal voltage Vb (V)>"
  Bus Selector3/3 -> Mux1/3  "<Terminal voltage Vc (V)>"
  Bus Selector3/1 -> Mux1/1  "<Terminal voltage Va (V)>"
  Mux1/1 -> To Workspace1/1, Scope5/1  "Vterminal"
  connections:
  Ground/LConn1 -- C1/RConn1 -- Simplified Synchronous Machine SI Units/LConn1
  P.O.R  and CTA/LConn1 -- parasitic resistive load/LConn1 -- Simplified Synchronous Machine SI Units/RConn1
  P.O.R  and CTA/LConn2 -- parasitic resistive load/LConn2 -- Simplified Synchronous Machine SI Units/RConn2
  P.O.R  and CTA/LConn3 -- parasitic resistive load/LConn3 -- Simplified Synchronous Machine SI Units/RConn3
  A/RConn1 -- P.O.R  and CTA/RConn1
  B/RConn1 -- P.O.R  and CTA/RConn2
  C/RConn1 -- P.O.R  and CTA/RConn3

== system power_aircraft_distribution_mexido_2016_V4/Primary Distribution (measurements & main contactor) ==
  note: Primary Distribution
  GLC control : Inport
  Contactor : Subsystem
  Current Measurement : powerlib/Measurements/Current Measurement  PhasorSimulation=off  OutputType=Complex  PSBequivalent=0
  Data Type Conversion : DataTypeConversion
  P.O.R  and CTA : powerlib/Measurements/Three-Phase V-I Measurement  VoltageMeasurement=phase-to-ground  SetLabelV=off  LabelV=Vabc  Vpu=off  VpuLL=off  CurrentMeasurement=yes  SetLabelI=off  LabelI=Iabc  Ipu=off  Pbase=100e6  Vbase=500e3  OutputType=Complex  PhasorSimulation=off  PSBequivalent=0
  Scope : Scope
  in_a : PMIOPort  Port=1  Side=Left
  in_b : PMIOPort  Port=2  Side=Left
  in_c : PMIOPort  Port=3  Side=Left
  out_a : PMIOPort  Port=4  Side=Right
  out_b : PMIOPort  Port=5  Side=Right
  out_c : PMIOPort  Port=6  Side=Right
  in_c1 : PMIOPort  Port=7  Side=Left
  out_c1 : PMIOPort  Port=8  Side=Right
  Vabc : Outport
  Iabc : Outport  Port=2
  wires:
  GLC control/1 -> Data Type Conversion/1
  P.O.R  and CTA/1 -> Vabc/1
  P.O.R  and CTA/2 -> Iabc/1
  Data Type Conversion/1 -> Contactor/1(com)
  Current Measurement/1 -> Scope/1
  connections:
  in_a/RConn1 -- P.O.R  and CTA/LConn1
  in_b/RConn1 -- P.O.R  and CTA/LConn2
  in_c/RConn1 -- P.O.R  and CTA/LConn3
  P.O.R  and CTA/RConn1 -- Contactor/LConn1
  P.O.R  and CTA/RConn2 -- Contactor/LConn2
  P.O.R  and CTA/RConn3 -- Contactor/LConn3
  Contactor/RConn1 -- out_a/RConn1
  out_b/RConn1 -- Contactor/RConn2
  Contactor/RConn3 -- out_c/RConn1
  Current Measurement/LConn1 -- in_c1/RConn1
  Current Measurement/RConn1 -- out_c1/RConn1

== system power_aircraft_distribution_mexido_2016_V4/Subsystem ==
  Iabc4 : Scope  NumInputPorts=2
  P.O.R  and CTA : powerlib/Measurements/Three-Phase V-I Measurement  VoltageMeasurement=phase-to-ground  SetLabelV=off  LabelV=Vabc  Vpu=off  VpuLL=off  CurrentMeasurement=yes  SetLabelI=off  LabelI=Iabc  Ipu=off  Pbase=100e6  Vbase=500e3  OutputType=Complex  PhasorSimulation=off  PSBequivalent=0
  Three-Phase Parallel RLC Load : powerlib/Elements/Three-Phase Parallel RLC Load  LConnTagsString=A|B|C  RConnTagsString=N  Configuration=Y (neutral)  NominalVoltage=115*sqrt(3)  Vabc=[1e3 1e3 1e3]  Vabcp=[1e3 1e3 1e3]  NominalFrequency=400  UnbalancedPower=off  ActivePower=3500  InductivePower=0  CapacitivePower=0  Pabc=[10e3 9e3 11e3]  QLabc=[100 90 110]  QCabc=[100 90 110]  Pabcp=[10e3 9e3 11e3]  QLabcp=[100 90 110]  QCabcp=[100 90 110]  Measurements=None  LoadType=constant Z
  va : PMIOPort  Port=1  Side=Left
  vb : PMIOPort  Port=2  Side=Left
  vc : PMIOPort  Port=3  Side=Left
  n : PMIOPort  Port=4  Side=Left
  wires:
  P.O.R  and CTA/1 -> Iabc4/1  "Vabc"
  P.O.R  and CTA/2 -> Iabc4/2  "Iabc"
  connections:
  n/RConn1 -- Three-Phase Parallel RLC Load/RConn1
  P.O.R  and CTA/RConn1 -- Three-Phase Parallel RLC Load/LConn1
  P.O.R  and CTA/RConn2 -- Three-Phase Parallel RLC Load/LConn2
  P.O.R  and CTA/RConn3 -- Three-Phase Parallel RLC Load/LConn3
  va/RConn1 -- P.O.R  and CTA/LConn1
  vb/RConn1 -- P.O.R  and CTA/LConn2
  vc/RConn1 -- P.O.R  and CTA/LConn3

== system power_aircraft_distribution_mexido_2016_V4/Subsystem1 ==
  Demux : Demux  Outputs=3
  Demux1 : Demux  Outputs=3
  Iabc4 : Scope  NumInputPorts=2
  Mux : Mux  Inputs=2
  P.O.R  and CTA : powerlib/Measurements/Three-Phase V-I Measurement  VoltageMeasurement=phase-to-ground  SetLabelV=off  LabelV=Vabc  Vpu=off  VpuLL=off  CurrentMeasurement=yes  SetLabelI=off  LabelI=Iabc  Ipu=off  Pbase=100e6  Vbase=500e3  OutputType=Complex  PhasorSimulation=off  PSBequivalent=0
  Series RLC Load : powerlib/Elements/Series RLC Load  LConnTagsString=a  RConnTagsString=__new0  NominalVoltage=115  NominalFrequency=400  ActivePower=1000  InductivePower=750  CapacitivePower=0  Setx0=off  InitialVoltage=0  SetiL0=off  InitialCurrent=0  Measurements=None  LoadType=constant Z
  Series RLC Load1 : powerlib/Elements/Series RLC Load  LConnTagsString=a  RConnTagsString=__new0  NominalVoltage=115  NominalFrequency=400  ActivePower=1000  InductivePower=750  CapacitivePower=0  Setx0=off  InitialVoltage=0  SetiL0=off  InitialCurrent=0  Measurements=None  LoadType=constant Z
  Series RLC Load2 : powerlib/Elements/Series RLC Load  LConnTagsString=a  RConnTagsString=__new0  NominalVoltage=115  NominalFrequency=400  ActivePower=1000  InductivePower=750  CapacitivePower=0  Setx0=off  InitialVoltage=0  SetiL0=off  InitialCurrent=0  Measurements=None  LoadType=constant Z
  va : PMIOPort  Port=1  Side=Left
  vb : PMIOPort  Port=2  Side=Left
  vc : PMIOPort  Port=3  Side=Left
  vn : PMIOPort  Port=4  Side=Left
  wires:
  P.O.R  and CTA/1 -> Demux/1  "Vabc"
  Demux/1 -> Mux/1  "Vabc"
  Demux1/1 -> Mux/2  "Iabc"
  P.O.R  and CTA/2 -> Iabc4/2, Demux1/1  "Iabc"
  Mux/1 -> Iabc4/1
  connections:
  va/RConn1 -- P.O.R  and CTA/LConn1
  vb/RConn1 -- P.O.R  and CTA/LConn2
  vc/RConn1 -- P.O.R  and CTA/LConn3
  vn/RConn1 -- Series RLC Load2/RConn1 -- Series RLC Load1/RConn1 -- Series RLC Load/RConn1
  P.O.R  and CTA/RConn1 -- Series RLC Load/LConn1
  Series RLC Load2/LConn1 -- P.O.R  and CTA/RConn3
  Series RLC Load1/LConn1 -- P.O.R  and CTA/RConn2

== system power_aircraft_distribution_mexido_2016_V4/Transformer and Rectifier Unit (TRU): 28 Vdc, 3920 W ==
  Current Measurement : powerlib/Measurements/Current Measurement  PhasorSimulation=off  OutputType=Complex  PSBequivalent=0
  Iabc1 : Scope  NumInputPorts=2
  Iabc4 : Scope  NumInputPorts=2
  P.O.R  and CTA : powerlib/Measurements/Three-Phase V-I Measurement  VoltageMeasurement=phase-to-ground  SetLabelV=off  LabelV=Vabc  Vpu=off  VpuLL=off  CurrentMeasurement=yes  SetLabelI=off  LabelI=Iabc  Ipu=off  Pbase=100e6  Vbase=500e3  OutputType=Complex  PhasorSimulation=off  PSBequivalent=0
  Series RLC Branch1 : powerlib/Elements/Series RLC Branch  LConnTagsString=__new0  RConnTagsString=__new0  BranchType=C  Resistance=1  Inductance=1e-3  SetiL0=off  InitialCurrent=0  Capacitance=10e-6  Setx0=off  InitialVoltage=0  Measurements=None
  Series RLC Branch2 : powerlib/Elements/Series RLC Branch  LConnTagsString=__new0  RConnTagsString=__new0  BranchType=L  Resistance=1  Inductance=0.1e-3  SetiL0=off  InitialCurrent=0  Capacitance=10e-6  Setx0=off  InitialVoltage=0  Measurements=None
  Series RLC Branch3 : powerlib/Elements/Series RLC Branch  LConnTagsString=__new0  RConnTagsString=__new0  BranchType=R  Resistance=1e3  Inductance=1e-3  SetiL0=off  InitialCurrent=0  Capacitance=1e-6  Setx0=off  InitialVoltage=0  Measurements=None
  Three-Phase Transformer (Three Windings) : powerlib/Elements/Three-Phase Transformer (Three Windings)  Winding1Connection=Yn  Winding2Connection=Delta (D1)  Winding3Connection=Y  CoreType=Three single-phase transformers  SetSaturation=off  Hysteresis=off  DataFile='hysteresis'  SetInitialFlux=off  Measurements=None  UNITS=pu  NominalPower=[ 20e3 , 400]  Winding1=[ 115*sqrt(3) , 0.002 , 0.08 ]  Winding2=[ 14.6/sqrt(2), 0.002 , 0.08 ]  Winding3=[ 14.6/sqrt(2) , 0.002 , 0.08 ]  Rm=800  Lm=800  L0=0.5  Saturation=[ 0,0 ; 0.0024,1.2 ; 1.0,1.52 ]  InitialFluxes=[0.8 -0.8 0.7]  MoreParameters=off  BreakLoop=off  DataType=off  TransfoNumber=1
  Universal Bridge : powerlib/Power Electronics/Universal Bridge  Arms=3  SnubberResistance=1e5  SnubberCapacitance=inf  Device=Diodes  Ron=1e-3  Lon=0  ForwardVoltages="[  0  0  ]"  ForwardVoltage=0  GTOparameters=[ 10e-6 , 20e-6 ]  IGBTparameters=[ 1e-6 , 2e-6 ]  Measurements=None  Measurements_2=None  converterType=Rectifier
  Universal Bridge1 : powerlib/Power Electronics/Universal Bridge  Arms=3  SnubberResistance=1e5  SnubberCapacitance=inf  Device=Diodes  Ron=1e-3  Lon=0  ForwardVoltages="[  0  0  ]"  ForwardVoltage=0  GTOparameters=[ 10e-6 , 20e-6 ]  IGBTparameters=[ 1e-6 , 2e-6 ]  Measurements=None  Measurements_2=None  converterType=Rectifier
  Voltage Measurement2 : powerlib/Measurements/Voltage Measurement  PhasorSimulation=off  OutputType=Complex  PSBequivalent=0
  A : PMIOPort  Port=1  Side=Left
  B : PMIOPort  Port=2  Side=Left
  + : PMIOPort  Port=3  Side=Right
  C : PMIOPort  Port=4  Side=Left
  N : PMIOPort  Port=5  Side=Left
  - : PMIOPort  Port=6  Side=Right
  wires:
  Voltage Measurement2/1 -> Iabc1/1  "Tensão Saída TRU"
  Current Measurement/1 -> Iabc1/2  "Corrente Saída TRU"
  P.O.R  and CTA/1 -> Iabc4/1  "Vabc"
  P.O.R  and CTA/2 -> Iabc4/2  "Iabc"
  connections:
  Three-Phase Transformer (Three Windings)/RConn1 -- Universal Bridge/LConn1
  Three-Phase Transformer (Three Windings)/RConn2 -- Universal Bridge/LConn2
  Three-Phase Transformer (Three Windings)/RConn3 -- Universal Bridge/LConn3
  Current Measurement/LConn1 -- Voltage Measurement2/LConn1 -- Series RLC Branch3/LConn1 -- Series RLC Branch2/LConn1 -- Series RLC Branch1/LConn1
  Three-Phase Transformer (Three Windings)/RConn4 -- Universal Bridge1/LConn1
  Three-Phase Transformer (Three Windings)/RConn5 -- Universal Bridge1/LConn2
  Three-Phase Transformer (Three Windings)/RConn6 -- Universal Bridge1/LConn3
  Universal Bridge1/RConn1 -- Universal Bridge/RConn2
  -/RConn1 -- Voltage Measurement2/LConn2 -- Series RLC Branch3/RConn1 -- Series RLC Branch1/RConn1 -- Universal Bridge1/RConn2
  Series RLC Branch2/RConn1 -- Universal Bridge/RConn1
  Current Measurement/RConn1 -- +/RConn1
  A/RConn1 -- P.O.R  and CTA/LConn1
  B/RConn1 -- P.O.R  and CTA/LConn2
  C/RConn1 -- P.O.R  and CTA/LConn3
  P.O.R  and CTA/RConn1 -- Three-Phase Transformer (Three Windings)/LConn1
  P.O.R  and CTA/RConn2 -- Three-Phase Transformer (Three Windings)/LConn2
  P.O.R  and CTA/RConn3 -- Three-Phase Transformer (Three Windings)/LConn3
  Three-Phase Transformer (Three Windings)/LConn4 -- N/RConn1

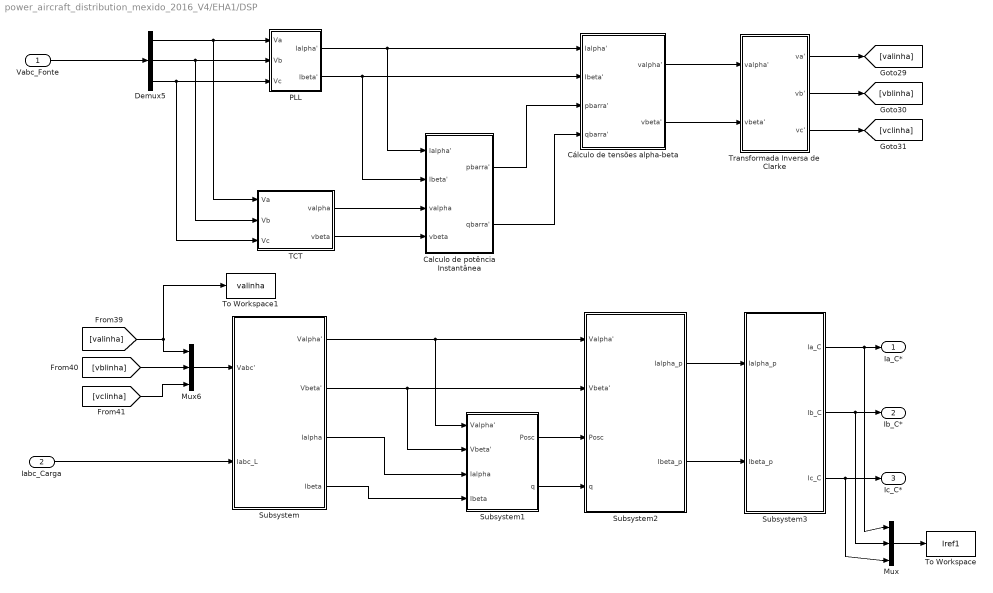
== system power_aircraft_distribution_mexido_2016_V4/EHA1/DSP ==
  Vabc_Fonte : Inport
  Iabc_Carga : Inport  Port=2
  Calculo de potência Instantânea : Subsystem
  Cálculo de tensões alpha-beta : Subsystem
  Demux5 : Demux  Outputs=3
  Mux : Mux  Inputs=3
  Mux6 : Mux  Inputs=3
  PLL : Subsystem
  Subsystem : Subsystem
  Subsystem1 : Subsystem
  Subsystem2 : Subsystem
  Subsystem3 : Subsystem
  TCT : Subsystem
  To Workspace : ToWorkspace  VariableName=Iref1  SaveFormat=Structure With Time  SampleTime=-1
  To Workspace1 : ToWorkspace  VariableName=valinha  SaveFormat=Structure With Time  SampleTime=-1
  Transformada Inversa de Clarke : Subsystem
  Ia_C* : Outport
  Ib_C* : Outport  Port=2
  Ic_C* : Outport  Port=3
  wires:
  Vabc_Fonte/1 -> Demux5/1
  Demux5/1 -> PLL/1(Va), TCT/1(Va)
  Demux5/2 -> PLL/2(Vb), TCT/2(Vb)
  Demux5/3 -> PLL/3(Vc), TCT/3(Vc)
  TCT/1(valpha) -> Calculo de potência Instantânea/3(valpha)
  TCT/2(vbeta) -> Calculo de potência Instantânea/4(vbeta)
  Calculo de potência Instantânea/2(qbarra') -> Cálculo de tensões alpha-beta/4(qbarra')
  PLL/1(Ialpha') -> Calculo de potência Instantânea/1(Ialpha'), Cálculo de tensões alpha-beta/1(Ialpha')
  PLL/2(Ibeta') -> Calculo de potência Instantânea/2(Ibeta'), Cálculo de tensões alpha-beta/2(Ibeta')
  Calculo de potência Instantânea/1(pbarra') -> Cálculo de tensões alpha-beta/3(pbarra')
  Cálculo de tensões alpha-beta/1(valpha') -> Transformada Inversa de Clarke/1(valpha')
  Cálculo de tensões alpha-beta/2(vbeta') -> Transformada Inversa de Clarke/2(vbeta')
  Transformada Inversa de Clarke/1(va') -> [valinha]
  Transformada Inversa de Clarke/2(vb') -> [vblinha]
  Transformada Inversa de Clarke/3(vc') -> [vclinha]
  [valinha] -> Mux6/1, To Workspace1/1
  [vblinha] -> Mux6/2
  [vclinha] -> Mux6/3
  Mux6/1 -> Subsystem/1(Vabc')
  Iabc_Carga/1 -> Subsystem/2(Iabc_L)
  Subsystem/1(Valpha') -> Subsystem1/1(Valpha'), Subsystem2/1(Valpha')
  Subsystem/3(Ialpha) -> Subsystem1/3(Ialpha)
  Subsystem/2(Vbeta') -> Subsystem1/2(Vbeta'), Subsystem2/2(Vbeta')
  Subsystem/4(Ibeta) -> Subsystem1/4(Ibeta)
  Subsystem1/1(Posc) -> Subsystem2/3(Posc)
  Subsystem1/2(q) -> Subsystem2/4(q)
  Subsystem3/1(Ia_C) -> Mux/1, Ia_C*/1
  Subsystem3/2(Ib_C) -> Mux/2, Ib_C*/1
  Subsystem3/3(Ic_C) -> Mux/3, Ic_C*/1
  Subsystem2/1(Ialpha_p) -> Subsystem3/1(Ialpha_p)
  Subsystem2/2(Ibeta_p) -> Subsystem3/2(Ibeta_p)
  Mux/1 -> To Workspace/1

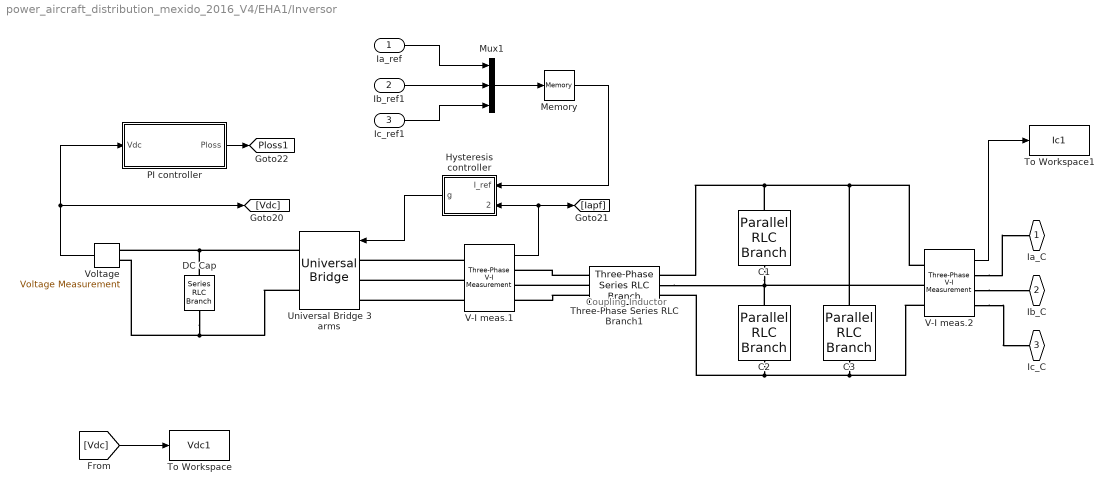
== system power_aircraft_distribution_mexido_2016_V4/EHA1/Inversor ==
  note: Coupling Inductor
  Ia_ref : Inport
  Ib_ref1 : Inport  Port=2
  Ic_ref1 : Inport  Port=3
  C1 : powerlib/Elements/Parallel RLC Branch  LConnTagsString=a  RConnTagsString=__new0  BranchType=C  Resistance=10e3  Inductance=1e-3  SetiL0=off  InitialCurrent=0  Capacitance=C  Setx0=off  InitialVoltage=0  Measurements=None
  C2 : powerlib/Elements/Parallel RLC Branch  LConnTagsString=a  RConnTagsString=__new0  BranchType=C  Resistance=10e3  Inductance=1e-3  SetiL0=off  InitialCurrent=0  Capacitance=C  Setx0=off  InitialVoltage=0  Measurements=None
  C3 : powerlib/Elements/Parallel RLC Branch  LConnTagsString=a  RConnTagsString=__new0  BranchType=C  Resistance=10e3  Inductance=1e-3  SetiL0=off  InitialCurrent=0  Capacitance=C  Setx0=off  InitialVoltage=0  Measurements=None
  DC Cap : powerlib/Elements/Series RLC Branch  LConnTagsString=__new0  RConnTagsString=__new0  BranchType=C  Resistance=1  Inductance=1e-3  SetiL0=off  InitialCurrent=0  Capacitance=200e-6  Setx0=off  InitialVoltage=350  Measurements=None
  Hysteresis controller : Subsystem
  Memory : Memory
  Mux1 : Mux  Inputs=3
  PI controller : Subsystem
  Three-Phase Series RLC Branch1 : powerlib/Elements/Three-Phase Series RLC Branch  LConnTagsString=A|B|C  RConnTagsString=A|B|C  BranchType=L  Resistance=1e9  Inductance=L  Capacitance=.2e-3  Measurements=None
  To Workspace : ToWorkspace  VariableName=Vdc1  SaveFormat=Structure With Time  SampleTime=-1
  To Workspace1 : ToWorkspace  VariableName=Ic1  SaveFormat=Structure With Time  SampleTime=-1
  Universal Bridge 3 arms : powerlib/Power Electronics/Universal Bridge  Arms=3  SnubberResistance=1e5  SnubberCapacitance=inf  Device=MOSFET / Diodes  Ron=1e-4  Lon=0  ForwardVoltages="[  1  1  ]"  ForwardVoltage=.8  GTOparameters=[ 10e-6 , 20e-6 ]  IGBTparameters=[ 1e-6 , 2e-6 ]  Measurements=All voltages and currents  Measurements_2=None  converterType=Rectifier
  V-I meas.1 : powerlib/Measurements/Three-Phase V-I Measurement  VoltageMeasurement=phase-to-phase  SetLabelV=on  LabelV=Vnm_EHA1  Vpu=off  VpuLL=off  CurrentMeasurement=yes  SetLabelI=off  LabelI=Iabc  Ipu=off  Pbase=100e6  Vbase=500e3  OutputType=Complex  PhasorSimulation=off  PSBequivalent=0
  V-I meas.2 : powerlib/Measurements/Three-Phase V-I Measurement  VoltageMeasurement=no  SetLabelV=off  LabelV=Vnm_EHA1  Vpu=off  VpuLL=off  CurrentMeasurement=yes  SetLabelI=off  LabelI=Iabc  Ipu=off  Pbase=100e6  Vbase=500e3  OutputType=Complex  PhasorSimulation=off  PSBequivalent=0
  Voltage : powerlib/Measurements/Voltage Measurement  PhasorSimulation=off  OutputType=Complex  PSBequivalent=0
  Ia_C : PMIOPort  Port=1  Side=Right
  Ib_C : PMIOPort  Port=2  Side=Right
  Ic_C : PMIOPort  Port=3  Side=Right
  tag scope: Ploss1=global
  wires:
  Voltage/1 -> [Vdc], PI controller/1(Vdc)
  PI controller/1(Ploss) -> [Ploss1]
  V-I meas.1/1 -> Hysteresis controller/2(I_meas), [Iapf]
  Mux1/1 -> Memory/1
  Hysteresis controller/1(g) -> Universal Bridge 3 arms/1
  Ia_ref/1 -> Mux1/1
  Ib_ref1/1 -> Mux1/2
  Ic_ref1/1 -> Mux1/3
  Memory/1 -> Hysteresis controller/1(I_ref)
  [Vdc] -> To Workspace/1
  V-I meas.2/1 -> To Workspace1/1
  connections:
  C3/RConn1 -- Three-Phase Series RLC Branch1/RConn3 -- C2/RConn1 -- V-I meas.2/LConn3
  Universal Bridge 3 arms/RConn1 -- DC Cap/LConn1 -- Voltage/LConn1
  DC Cap/RConn1 -- Voltage/LConn2 -- Universal Bridge 3 arms/RConn2
  Three-Phase Series RLC Branch1/LConn2 -- V-I meas.1/RConn2
  V-I meas.1/LConn1 -- Universal Bridge 3 arms/LConn1
  Three-Phase Series RLC Branch1/LConn1 -- V-I meas.1/RConn1
  V-I meas.1/LConn2 -- Universal Bridge 3 arms/LConn2
  Three-Phase Series RLC Branch1/LConn3 -- V-I meas.1/RConn3
  V-I meas.1/LConn3 -- Universal Bridge 3 arms/LConn3
  C3/LConn1 -- V-I meas.2/LConn1 -- C1/LConn1 -- Three-Phase Series RLC Branch1/RConn1
  Three-Phase Series RLC Branch1/RConn2 -- V-I meas.2/LConn2 -- C2/LConn1 -- C1/RConn1
  V-I meas.2/RConn1 -- Ia_C/RConn1
  V-I meas.2/RConn2 -- Ib_C/RConn1
  V-I meas.2/RConn3 -- Ic_C/RConn1

== system power_aircraft_distribution_mexido_2016_V4/EHA1/Signal Builder ==
  Demux : Demux  Tag=STV Demux  Outputs=1
  FromWs : FromWorkspace  Tag=STV FromWs  VariableName=tuvar  SampleTime=0
      SigBuilderData=|
      | common.afterFinalStr = 'Extrapolate'
      | common.sampleTime = 0
      | dataSet.timeRange = [72.8 73.9160839161]
      | dataSet.name = 'Imported_Group 1'
      | sbobj.Name = 'Signal Builder'
      | sbobj.Groups.Name = 'Imported_Group 1'
      | sbobj.Groups.Signals.Name = 'var'
      | sbobj.Groups.Signals.XData = [72.8 72.8335664336 72.8671328671 72.8951048951 72.9202797203 72.9398601399 72.965034965 72.9818181818 72.9958041958 73.0097902098 73.0125874126 73.0181818182 73.0237762238 73.0293706294 73.0377622378 73.0433566434 73.048951049 73.0601398601 73.0657342657 73.0741258741 73.0853146853 73.0965034965 73.1104895105 73.1244755245 73.1356643357 73.1552447552 73.1832167832 73.1888111888 73.2111888112 73.227972028 73.2475524476 73.2615384615 73.2643356643 73.2699300699 73.2727272727 73.2755244755 73.2783216783 73.2811188811 73.2839160839 73.2895104895 73.2979020979 73.3090909091 73.3230769231 73.3454545455 73.3678321678 73.393006993 73.4181818182 73.434965035 73.4573426573 73.4825174825 73.5048951049 73.5216783217 73.5440559441 73.5664335664 73.5832167832 73.6027972028 73.627972028 73.6531468531 73.6811188811 73.7006993007 73.7286713287 73.751048951 73.7734265734 73.7902097902 73.8097902098 73.8293706294 73.8517482517 73.8657342657 73.8853146853 73.9048951049 73.9160839161]
      | sbobj.Groups.Signals.YData = [-0.319653102263 -0.326498736815 -0.333344371367 -0.339049066827 -0.34418329274 -0.348176579562 -0.353310805476 -0.356733622752 -0.359585970482 1.59541316359 6.48947139854 11.0566505836 17.2553726702 21.496243275 26.7154691512 31.2826483363 35.5235189411 39.7632486068 44.6567363722 49.8759622484 54.4420004944 59.0080387404 63.8998150972 69.1179000342 65.1999151925 63.2380704238 62.2534399875 60.9470647272 61.5951181314 60.6127695732 59.6298505455 59.3006896175 49.8371703193 39.0678462303 24.0570810669 13.9409446081 11.6562140765 9.69779212512 8.71829591467 6.10668633318 4.79974060335 3.49222440397 2.18413773504 1.52695681807 0.869775901102 0.864641675188 0.859507449274 1.1823932123 1.17782945593 1.49900381032 1.82074863425 1.81732581697 1.4864534803 1.48188972394 1.15215832636 0.82185645924 0.490413653026 0.485279427112 0.479574731653 0.149272864531 0.143568169071 -0.187304167596 -0.191867923964 -0.52159932154 -0.525592608362 -0.529585895183 -0.534149651551 -0.537001999281 -0.540995286103 -0.544988572925 -0.547270451109]
      | sbobj.Groups.TimeRange = [72.8 73.9160839161]
  var : Outport
  wires:
  Demux/1 -> var/1
  FromWs/1 -> Demux/1

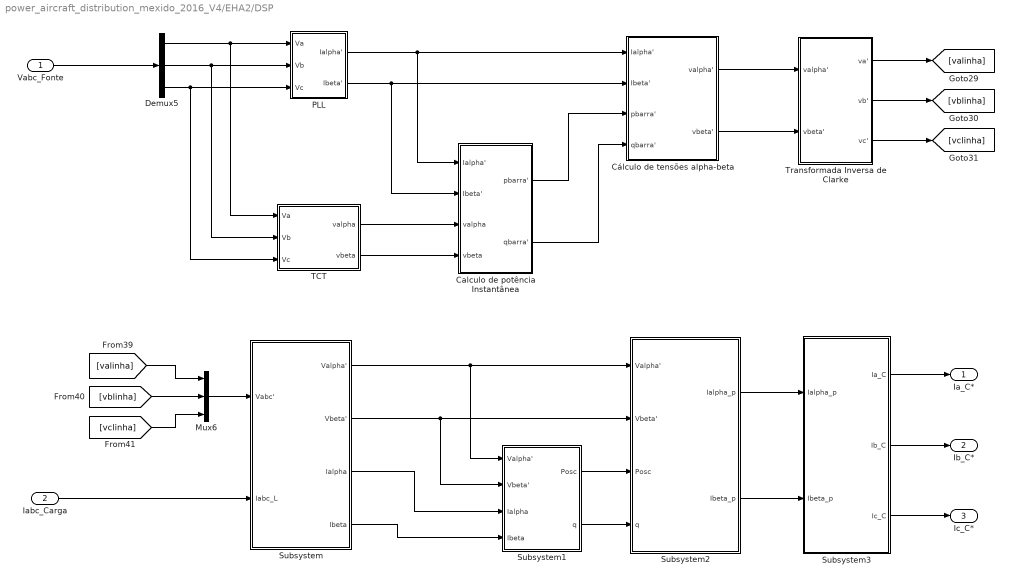
== system power_aircraft_distribution_mexido_2016_V4/EHA2/DSP ==
  Vabc_Fonte : Inport
  Iabc_Carga : Inport  Port=2
  Calculo de potência Instantânea : Subsystem
  Cálculo de tensões alpha-beta : Subsystem
  Demux5 : Demux  Outputs=3
  Mux6 : Mux  Inputs=3
  PLL : Subsystem
  Subsystem : Subsystem
  Subsystem1 : Subsystem
  Subsystem2 : Subsystem
  Subsystem3 : Subsystem
  TCT : Subsystem
  Transformada Inversa de Clarke : Subsystem
  Ia_C* : Outport
  Ib_C* : Outport  Port=2
  Ic_C* : Outport  Port=3
  wires:
  Vabc_Fonte/1 -> Demux5/1
  Demux5/1 -> PLL/1(Va), TCT/1(Va)
  Demux5/2 -> PLL/2(Vb), TCT/2(Vb)
  Demux5/3 -> PLL/3(Vc), TCT/3(Vc)
  TCT/1(valpha) -> Calculo de potência Instantânea/3(valpha)
  TCT/2(vbeta) -> Calculo de potência Instantânea/4(vbeta)
  Calculo de potência Instantânea/2(qbarra') -> Cálculo de tensões alpha-beta/4(qbarra')
  PLL/1(Ialpha') -> Calculo de potência Instantânea/1(Ialpha'), Cálculo de tensões alpha-beta/1(Ialpha')
  PLL/2(Ibeta') -> Calculo de potência Instantânea/2(Ibeta'), Cálculo de tensões alpha-beta/2(Ibeta')
  Calculo de potência Instantânea/1(pbarra') -> Cálculo de tensões alpha-beta/3(pbarra')
  Cálculo de tensões alpha-beta/1(valpha') -> Transformada Inversa de Clarke/1(valpha')
  Cálculo de tensões alpha-beta/2(vbeta') -> Transformada Inversa de Clarke/2(vbeta')
  Transformada Inversa de Clarke/1(va') -> [valinha]
  Transformada Inversa de Clarke/2(vb') -> [vblinha]
  Transformada Inversa de Clarke/3(vc') -> [vclinha]
  [valinha] -> Mux6/1
  [vblinha] -> Mux6/2
  [vclinha] -> Mux6/3
  Mux6/1 -> Subsystem/1(Vabc')
  Iabc_Carga/1 -> Subsystem/2(Iabc_L)
  Subsystem/1(Valpha') -> Subsystem1/1(Valpha'), Subsystem2/1(Valpha')
  Subsystem/3(Ialpha) -> Subsystem1/3(Ialpha)
  Subsystem/2(Vbeta') -> Subsystem1/2(Vbeta'), Subsystem2/2(Vbeta')
  Subsystem/4(Ibeta) -> Subsystem1/4(Ibeta)
  Subsystem1/1(Posc) -> Subsystem2/3(Posc)
  Subsystem1/2(q) -> Subsystem2/4(q)
  Subsystem3/1(Ia_C) -> Ia_C*/1
  Subsystem3/2(Ib_C) -> Ib_C*/1
  Subsystem3/3(Ic_C) -> Ic_C*/1
  Subsystem2/1(Ialpha_p) -> Subsystem3/1(Ialpha_p)
  Subsystem2/2(Ibeta_p) -> Subsystem3/2(Ibeta_p)
